simulink model "mapp_4_fir_4_str"  (R2018b)
settings: Solver=ode45  StartTime=0.0  StopTime=200  RelTol=1e-3  EnableMultiTasking=on
undefined symbols (not defined in the file or in its folder): CMD_ci_Re_0, CMD_ci_Re_21, CMD_ci_str_0, CMD_ci_str_1, CMD_ci_str_10, CMD_ci_str_11, CMD_ci_str_12, CMD_ci_str_13, CMD_ci_str_14, CMD_ci_str_15, CMD_ci_str_16, CMD_ci_str_17, CMD_ci_str_18, CMD_ci_str_19, CMD_ci_str_2, CMD_ci_str_20, CMD_ci_str_21, CMD_ci_str_3, CMD_ci_str_4, CMD_ci_str_5, CMD_ci_str_6, CMD_ci_str_7, CMD_ci_str_8, CMD_ci_str_9, CMD_decr_0, CMD_deka_down, CMD_deka_up, CMD_fb, CMD_FB_mult, CMD_Firprg_0, CMD_Firprg_1, CMD_gain, CMD_ind_mult, CMD_ind_mult_1, CMD_ind_mult_2, CMD_ind_mult_3, CMD_ind_mult_4, CMD_ind_stuk, CMD_ind_vol, CMD_ind_vol_1, CMD_ind_vol_2, CMD_ind_vol_3, CMD_ind_vol_4, CMD_init_dac, CMD_init_sw, CMD_molot_string, CMD_nl, CMD_nl_sl, CMD_omega_0, CMD_out_vol, CMD_param_0, CMD_param_5, CMD_pedal, CMD_reset, CMD_rst, CMD_shape_0, CMD_step_down, CMD_step_up, CMD_str_svertk, ind_mult_0 ... (+10)
libraries: xbsIndex_r4 x3300
(part 5 of 16)

== system mapp_4_fir_4_str/MUX0/ci_re_21 ==
  addr : Inport
  m_data : Inport  Port=2
  m_addr : Inport  Port=3
  m_en : Inport  Port=4
  Convert2 : xbsIndex_r4/Convert  gui_display_data_type=Floating-point  arith_type=Floating-point  n_bits=16  bin_pt=14  float_type=Single  exp_bits=8  fraction_bits=24  quantization=Truncate  overflow=Wrap  en=off  latency=6  pipeline=off  dbl_ovrd=off  block_type=convert
  Delay{1..5} (5 alike) : xbsIndex_r4/Delay  rst=off  infoeditControl=Selection of Reset will increase slice count due to use of real FFs and instead of SRLs  en=off  latency=1  reg_retiming=off  dbl_ovrd=off  block_type=delay
  Mux1 : xbsIndex_r4/Mux  inputs=2  en=off  latency=0  precision=Full  arith_type=Unsigned  n_bits=16  bin_pt=14  quantization=Truncate  overflow=Wrap  dbl_ovrd=off  block_type=mux
  Reinterpret9 : xbsIndex_r4/Reinterpret  force_arith_type=on  arith_type=Floating-point  force_bin_pt=on  bin_pt=24  block_type=reinterpret
  Relational14 : xbsIndex_r4/Relational  mode=a=b  op_type=Bool  en=off  latency=0  dbl_ovrd=off  block_type=relational
  Single Port RAM2 : xbsIndex_r4/Single Port RAM  depth=1024  initVector=Res1  distributed_mem=Block RAM  write_mode=Read After Write  rst=off  init_reg=0  en=off  latency=1  optimize=Area  dbl_ovrd=off  block_type=spram
  re_0 : xbsIndex_r4/Constant  const=CMD_ci_Re_21  gui_display_data_type=Fixed-point  arith_type=Unsigned  n_bits=8  bin_pt=0  preci_type=Single  exp_width=8  frac_width=24  explicit_period=on  period=1  equ=P=C  opselect=C  inp2=PCIN>>17  opr=+  inp1=P  carry=CIN  dbl_ovrd=off  block_type=constant
      settings: block_version=VER_STRING_GOES_HERE
  Out : Outport
  wires:
  Delay5/1 -> Single Port RAM2/3, Mux1/1
  Delay1/1 -> Single Port RAM2/2
  Delay4/1 -> Out/1
  Single Port RAM2/1 -> Delay2/1
  Convert2/1 -> Delay4/1
  Delay2/1 -> Reinterpret9/1
  Reinterpret9/1 -> Delay3/1
  Delay3/1 -> Convert2/1
  Mux1/1 -> Single Port RAM2/1
  re_0/1 -> Relational14/2
  Relational14/1 -> Delay5/1
  addr/1 -> Mux1/2
  m_en/1 -> Relational14/1
  m_addr/1 -> Mux1/3
  m_data/1 -> Delay1/1

== system mapp_4_fir_4_str/Mid_Graph2/Exp ==
  note: w5
  Addr_ind_vol : Inport
  Force_vol_sel : Inport  Port=2
  Addr0 : Inport  Port=3
  m_data : Inport  Port=4
  m_addr : Inport  Port=5
  m_en : Inport  Port=6
  Constant3 : xbsIndex_r4/Constant  const=0  gui_display_data_type=Fixed-point  arith_type=Unsigned  n_bits=7  bin_pt=0  preci_type=Single  exp_width=8  frac_width=24  explicit_period=on  period=1  equ=P=C  opselect=C  inp2=PCIN>>17  opr=+  inp1=P  carry=CIN  dbl_ovrd=off  block_type=constant
      settings: block_version=VER_STRING_GOES_HERE
  Convert1 : xbsIndex_r4/Convert  gui_display_data_type=Floating-point  arith_type=Floating-point  n_bits=16  bin_pt=14  float_type=Single  exp_bits=8  fraction_bits=24  quantization=Truncate  overflow=Wrap  en=off  latency=0  pipeline=off  dbl_ovrd=off  block_type=convert
  Convert2 : xbsIndex_r4/Convert  gui_display_data_type=Floating-point  arith_type=Floating-point  n_bits=16  bin_pt=14  float_type=Single  exp_bits=8  fraction_bits=24  quantization=Truncate  overflow=Wrap  en=off  latency=0  pipeline=off  dbl_ovrd=off  block_type=convert
  Convert6 : xbsIndex_r4/Convert  gui_display_data_type=Floating-point  arith_type=Floating-point  n_bits=16  bin_pt=14  float_type=Single  exp_bits=8  fraction_bits=24  quantization=Truncate  overflow=Wrap  en=off  latency=0  pipeline=off  dbl_ovrd=off  block_type=convert
  Convert9 : xbsIndex_r4/Convert  gui_display_data_type=Fixed-point  arith_type=Unsigned  n_bits=24  bin_pt=0  float_type=Single  exp_bits=8  fraction_bits=24  quantization=Truncate  overflow=Wrap  en=off  latency=0  pipeline=off  dbl_ovrd=off  block_type=convert
  Mult : xbsIndex_r4/Mult  precision=Full  arith_type="Signed  (2's comp)"  n_bits=16  bin_pt=14  quantization=Truncate  overflow=Wrap  en=off  latency=6  use_behavioral_HDL=off  opt=Speed  use_embedded=on  optimum_pipeline=off  pipeline=on  dbl_ovrd=off  use_rpm=on  placement_style=Triangular  block_type=mult
  Mult1 : xbsIndex_r4/Mult  precision=Full  arith_type="Signed  (2's comp)"  n_bits=16  bin_pt=14  quantization=Truncate  overflow=Wrap  en=off  latency=6  use_behavioral_HDL=off  opt=Speed  use_embedded=on  optimum_pipeline=off  pipeline=on  dbl_ovrd=off  use_rpm=on  placement_style=Triangular  block_type=mult
  Relational16 : xbsIndex_r4/Relational  mode=a=b  op_type=Bool  en=off  latency=0  dbl_ovrd=off  block_type=relational
  Scope2 : Scope  NumInputPorts=9
  Scope3 : Scope  NumInputPorts=9
  const : xbsIndex_r4/Constant  const=0  gui_display_data_type=Fixed-point  arith_type=Unsigned  n_bits=7  bin_pt=0  preci_type=Single  exp_width=8  frac_width=24  explicit_period=on  period=1  equ=P=C  opselect=C  inp2=PCIN>>17  opr=+  inp1=P  carry=CIN  dbl_ovrd=off  block_type=constant
      settings: block_version=VER_STRING_GOES_HERE
  exp-mashinka : Subsystem
  ind_tails : Subsystem
  ind_vol : Subsystem
  z1 : xbsIndex_r4/Delay  rst=off  infoeditControl=Selection of Reset will increase slice count due to use of real FFs and instead of SRLs  en=off  latency=66  reg_retiming=on  dbl_ovrd=off  block_type=delay
      settings: block_version=8.2-EVAL
  z{2..3,5..7} (5 alike) : xbsIndex_r4/Delay  rst=off  infoeditControl=Selection of Reset will increase slice count due to use of real FFs and instead of SRLs  en=off  latency=1  reg_retiming=on  dbl_ovrd=off  block_type=delay
      settings: block_version=8.2-EVAL
  z4 : xbsIndex_r4/Delay  rst=off  infoeditControl=Selection of Reset will increase slice count due to use of real FFs and instead of SRLs  en=off  latency=66 + 7  reg_retiming=on  dbl_ovrd=off  block_type=delay
      settings: block_version=8.2-EVAL
  z53 : xbsIndex_r4/Delay  rst=off  infoeditControl=Selection of Reset will increase slice count due to use of real FFs and instead of SRLs  en=off  latency=9  reg_retiming=on  dbl_ovrd=off  block_type=delay
      settings: block_version=8.2-EVAL
  z8 : xbsIndex_r4/Delay  rst=off  infoeditControl=Selection of Reset will increase slice count due to use of real FFs and instead of SRLs  en=off  latency=2  reg_retiming=on  dbl_ovrd=off  block_type=delay
      settings: block_version=8.2-EVAL
  FF : Outport
  Stuk : Outport  Port=2
  wires:
  z7/1 -> Mult1/1
  z6/1 -> Stuk/1
  Mult1/1 -> z6/1
  z5/1 -> Mult1/2
  ind_tails/1(Out1) -> z4/1
  z4/1 -> z5/1
  z3/1 -> FF/1
  Mult/1 -> z7/1, Convert2/1, z3/1
  Convert2/1 -> Scope3/3
  Convert1/1 -> Scope3/2
  exp-mashinka/1(Out) -> Convert6/1, Mult/1
  z2/1 -> Mult/2, Convert1/1
  z1/1 -> z2/1
  Convert6/1 -> Scope3/1
  ind_vol/1(Out1) -> z1/1
  Relational16/1 -> z53/1
  const/1 -> Relational16/2
  m_addr/1 -> exp-mashinka/3(m_addr), ind_vol/3(m_addr), ind_tails/3(m_addr)
  m_data/1 -> Convert9/1, exp-mashinka/2(m_data), ind_vol/2(dat_in), ind_tails/2(dat_in)
  m_en/1 -> exp-mashinka/4(m_en), ind_vol/4(m_en), ind_tails/4(m_en)
  z8/1 -> exp-mashinka/1(Force_vol), ind_vol/5(force_vol), ind_tails/5(force_vol)
  Addr_ind_vol/1 -> exp-mashinka/5(Addr_ind_vol), ind_vol/1(addr_ind_vol), ind_tails/1(addr_ind_vol), Scope2/1
  Addr0/1 -> exp-mashinka/6(Addr_sync), Scope2/3
  Force_vol_sel/1 -> Relational16/1, Scope2/2, z8/1

== system mapp_4_fir_4_str/Mid_Graph2/ind_mult ==
  addr : Inport
  dat_in : Inport  Port=2
  addr_prg : Inport  Port=3
  prg_en : Inport  Port=4
  force_vol : Inport  Port=5
  AddSub5 : xbsIndex_r4/AddSub  mode=Subtraction  use_carryin=off  use_carryout=off  en=off  latency=2  precision=Full  arith_type="Signed  (2's comp)"  n_bits=24  bin_pt=0  quantization=Truncate  overflow=Wrap  use_behavioral_HDL=off  hw_selection=Fabric  pipelined=off  dbl_ovrd=off  block_type=addsub
  AddSub6 : xbsIndex_r4/AddSub  mode=Addition  use_carryin=off  use_carryout=off  en=off  latency=2  precision=Full  arith_type=Unsigned  n_bits=24  bin_pt=0  quantization=Truncate  overflow=Wrap  use_behavioral_HDL=off  hw_selection=Fabric  pipelined=off  dbl_ovrd=off  block_type=addsub
  Constant : xbsIndex_r4/Constant  const=4  gui_display_data_type=Fixed-point  arith_type=Unsigned  n_bits=3  bin_pt=0  preci_type=Single  exp_width=8  frac_width=24  explicit_period=off  period=1  equ=P=C  opselect=C  inp2=PCIN>>17  opr=+  inp1=P  carry=CIN  dbl_ovrd=off  block_type=constant
  Constant1 : xbsIndex_r4/Constant  const=0  gui_display_data_type=Fixed-point  arith_type=Unsigned  n_bits=24  bin_pt=0  preci_type=Single  exp_width=8  frac_width=24  explicit_period=on  period=1  equ=P=C  opselect=C  inp2=PCIN>>17  opr=+  inp1=P  carry=CIN  dbl_ovrd=off  block_type=constant
      settings: block_version=VER_STRING_GOES_HERE
  Constant10 : xbsIndex_r4/Constant  const=0  gui_display_data_type=Fixed-point  arith_type=Unsigned  n_bits=24  bin_pt=0  preci_type=Single  exp_width=8  frac_width=24  explicit_period=on  period=1  equ=P=C  opselect=C  inp2=PCIN>>17  opr=+  inp1=P  carry=CIN  dbl_ovrd=off  block_type=constant
      settings: block_version=VER_STRING_GOES_HERE
  Constant2 : xbsIndex_r4/Constant  const=4  gui_display_data_type=Fixed-point  arith_type=Unsigned  n_bits=3  bin_pt=0  preci_type=Single  exp_width=8  frac_width=24  explicit_period=on  period=1  equ=P=C  opselect=C  inp2=PCIN>>17  opr=+  inp1=P  carry=CIN  dbl_ovrd=off  block_type=constant
      settings: block_version=VER_STRING_GOES_HERE
  Constant3 : xbsIndex_r4/Constant  const=3  gui_display_data_type=Fixed-point  arith_type=Unsigned  n_bits=3  bin_pt=0  preci_type=Single  exp_width=8  frac_width=24  explicit_period=off  period=1  equ=P=C  opselect=C  inp2=PCIN>>17  opr=+  inp1=P  carry=CIN  dbl_ovrd=off  block_type=constant
  Constant4 : xbsIndex_r4/Constant  const=2  gui_display_data_type=Fixed-point  arith_type=Unsigned  n_bits=3  bin_pt=0  preci_type=Single  exp_width=8  frac_width=24  explicit_period=off  period=1  equ=P=C  opselect=C  inp2=PCIN>>17  opr=+  inp1=P  carry=CIN  dbl_ovrd=off  block_type=constant
  Constant5 : xbsIndex_r4/Constant  const=1  gui_display_data_type=Fixed-point  arith_type=Unsigned  n_bits=3  bin_pt=0  preci_type=Single  exp_width=8  frac_width=24  explicit_period=off  period=1  equ=P=C  opselect=C  inp2=PCIN>>17  opr=+  inp1=P  carry=CIN  dbl_ovrd=off  block_type=constant
  Constant6 : xbsIndex_r4/Constant  const=0  gui_display_data_type=Fixed-point  arith_type=Unsigned  n_bits=3  bin_pt=0  preci_type=Single  exp_width=8  frac_width=24  explicit_period=off  period=1  equ=P=C  opselect=C  inp2=PCIN>>17  opr=+  inp1=P  carry=CIN  dbl_ovrd=off  block_type=constant
  Convert5 : xbsIndex_r4/Convert  gui_display_data_type=Fixed-point  arith_type=Unsigned  n_bits=3  bin_pt=0  float_type=Single  exp_bits=8  fraction_bits=24  quantization=Truncate  overflow=Wrap  en=off  latency=0  pipeline=off  dbl_ovrd=off  block_type=convert
  Logical{,1..4} (5 alike) : xbsIndex_r4/Logical  logical_function=AND  inputs=2  en=off  latency=1  precision=Full  arith_type=Unsigned  n_bits=16  bin_pt=0  align_bp=on  dbl_ovrd=off  block_type=logical
  Mult3 : xbsIndex_r4/Mult  precision=Full  arith_type="Signed  (2's comp)"  n_bits=16  bin_pt=14  quantization=Truncate  overflow=Wrap  en=off  latency=3  use_behavioral_HDL=off  opt=Speed  use_embedded=on  optimum_pipeline=off  pipeline=on  dbl_ovrd=off  use_rpm=on  placement_style=Triangular  block_type=mult
  Mux{1,10..14} (6 alike) : xbsIndex_r4/Mux  inputs=2  en=off  latency=0  precision=Full  arith_type=Unsigned  n_bits=16  bin_pt=14  quantization=Truncate  overflow=Wrap  dbl_ovrd=off  block_type=mux
  Mux2 : xbsIndex_r4/Mux  inputs=5  en=off  latency=1  precision=Full  arith_type=Unsigned  n_bits=16  bin_pt=14  quantization=Truncate  overflow=Wrap  dbl_ovrd=off  block_type=mux
  Mux3 : xbsIndex_r4/Mux  inputs=5  en=off  latency=1  precision=Full  arith_type=Unsigned  n_bits=16  bin_pt=14  quantization=Truncate  overflow=Wrap  dbl_ovrd=off  block_type=mux
  RSlice1 : xbsIndex_r4/Slice  nbits=3  boolean_output=off  mode=Upper Bit Location + Width  bit1=0  base1=MSB of Input  bit0=0  base0=LSB of Input  dbl_ovrd=off  block_type=slice
      settings: block_version=VER_STRING_GOES_HERE
  RSlice7 : xbsIndex_r4/Slice  nbits=7  boolean_output=off  mode=Lower Bit Location + Width  bit1=0  base1=MSB of Input  bit0=0  base0=LSB of Input  dbl_ovrd=off  block_type=slice
      settings: block_version=VER_STRING_GOES_HERE
  Relational{1..5,16..17} (7 alike) : xbsIndex_r4/Relational  mode=a=b  op_type=Bool  en=off  latency=0  dbl_ovrd=off  block_type=relational
  Scope1 : Scope  NumInputPorts=8
  Scope2 : Scope  NumInputPorts=10
  Scope3 : Scope  NumInputPorts=10
  Scope4 : Scope  NumInputPorts=10
  Shift2 : xbsIndex_r4/Shift  shift_dir=Right  shift_bits=5  en=off  latency=0  precision=Full  arith_type="Signed  (2's comp)"  n_bits=16  bin_pt=14  quantization=Truncate  overflow=Wrap  dbl_ovrd=off  block_type=shift
  Single Port RAM5 : xbsIndex_r4/Single Port RAM  depth=96  initVector=ind_mult_4*ind_mult_multiplier  distributed_mem=Block RAM  write_mode=Read After Write  rst=off  init_reg=0  en=off  latency=1  optimize=Area  dbl_ovrd=off  block_type=spram
  Single Port RAM6 : xbsIndex_r4/Single Port RAM  depth=96  initVector=ind_mult_3*ind_mult_multiplier  distributed_mem=Block RAM  write_mode=Read After Write  rst=off  init_reg=0  en=off  latency=1  optimize=Area  dbl_ovrd=off  block_type=spram
  Single Port RAM7 : xbsIndex_r4/Single Port RAM  depth=96  initVector=ind_mult_2*ind_mult_multiplier  distributed_mem=Block RAM  write_mode=Read After Write  rst=off  init_reg=0  en=off  latency=1  optimize=Area  dbl_ovrd=off  block_type=spram
  Single Port RAM8 : xbsIndex_r4/Single Port RAM  depth=96  initVector=ind_mult_1*ind_mult_multiplier  distributed_mem=Block RAM  write_mode=Read After Write  rst=off  init_reg=0  en=off  latency=1  optimize=Area  dbl_ovrd=off  block_type=spram
  Single Port RAM9 : xbsIndex_r4/Single Port RAM  depth=96  initVector=ind_mult_0*ind_mult_multiplier  distributed_mem=Block RAM  write_mode=Read After Write  rst=off  init_reg=0  en=off  latency=1  optimize=Area  dbl_ovrd=off  block_type=spram
  Slice1 : xbsIndex_r4/Slice  nbits=5  boolean_output=off  mode=Lower Bit Location + Width  bit1=0  base1=LSB of Input  bit0=0  base0=LSB of Input  dbl_ovrd=off  block_type=slice
  Slice3 : xbsIndex_r4/Slice  nbits=2  boolean_output=off  mode=Upper Bit Location + Width  bit1=0  base1=MSB of Input  bit0=0  base0=LSB of Input  dbl_ovrd=off  block_type=slice
  const : xbsIndex_r4/Constant  const=0  gui_display_data_type=Fixed-point  arith_type=Unsigned  n_bits=7  bin_pt=0  preci_type=Single  exp_width=8  frac_width=24  explicit_period=on  period=1  equ=P=C  opselect=C  inp2=PCIN>>17  opr=+  inp1=P  carry=CIN  dbl_ovrd=off  block_type=constant
      settings: block_version=VER_STRING_GOES_HERE
  ind_mult : xbsIndex_r4/Constant  const=CMD_ind_mult  gui_display_data_type=Fixed-point  arith_type=Unsigned  n_bits=8  bin_pt=0  preci_type=Single  exp_width=8  frac_width=24  explicit_period=on  period=1  equ=P=C  opselect=C  inp2=PCIN>>17  opr=+  inp1=P  carry=CIN  dbl_ovrd=off  block_type=constant
      settings: block_version=VER_STRING_GOES_HERE
  x : xbsIndex_r4/Constant  const=8000000  gui_display_data_type=Fixed-point  arith_type=Unsigned  n_bits=24  bin_pt=0  preci_type=Single  exp_width=8  frac_width=24  explicit_period=on  period=1  equ=P=C  opselect=C  inp2=PCIN>>17  opr=+  inp1=P  carry=CIN  dbl_ovrd=off  block_type=constant
      settings: block_version=VER_STRING_GOES_HERE
  z1 : xbsIndex_r4/Delay  rst=off  infoeditControl=Selection of Reset will increase slice count due to use of real FFs and instead of SRLs  en=off  latency=3  reg_retiming=on  dbl_ovrd=off  block_type=delay
      settings: block_version=8.2-EVAL
  z{2,5..13,15} (11 alike) : xbsIndex_r4/Delay  rst=off  infoeditControl=Selection of Reset will increase slice count due to use of real FFs and instead of SRLs  en=off  latency=1  reg_retiming=on  dbl_ovrd=off  block_type=delay
      settings: block_version=8.2-EVAL
  z14 : xbsIndex_r4/Delay  rst=off  infoeditControl=Selection of Reset will increase slice count due to use of real FFs and instead of SRLs  en=off  latency=2  reg_retiming=on  dbl_ovrd=off  block_type=delay
      settings: block_version=8.2-EVAL
  z3 : xbsIndex_r4/Delay  rst=off  infoeditControl=Selection of Reset will increase slice count due to use of real FFs and instead of SRLs  en=off  latency=4  reg_retiming=on  dbl_ovrd=off  block_type=delay
      settings: block_version=8.2-EVAL
  z4 : xbsIndex_r4/Delay  rst=off  infoeditControl=Selection of Reset will increase slice count due to use of real FFs and instead of SRLs  en=off  latency=2  reg_retiming=on  dbl_ovrd=off  block_type=delay
      settings: block_version=8.2-EVAL
  Out1 : Outport
  wires:
  z1/1 -> Mult3/2, Scope1/5
  Mux1/1 -> Scope3/1, Mux2/1, Mux3/1
  z15/1 -> Mux3/2
  z13/1 -> Scope3/2, Mux2/2, Mux3/3
  z12/1 -> Mux3/4, Scope3/3, Mux2/3
  z11/1 -> Scope3/4, Mux2/4, Mux3/5
  z10/1 -> Scope3/5, Mux2/5
  AddSub6/1 -> Out1/1, Scope1/8
  z3/1 -> AddSub6/2, Scope1/7
  z14/1 -> z3/1
  z2/1 -> AddSub6/1, Scope1/6
  Mult3/1 -> z2/1
  Slice1/1 -> z1/1
  Shift2/1 -> Mult3/1, Scope1/4
  AddSub5/1 -> Shift2/1, Scope1/3
  Mux3/1 -> AddSub5/2, Scope1/2, Scope3/7, z14/1
  Mux2/1 -> AddSub5/1, Scope1/1, Scope3/6
  Constant1/1 -> Mux3/6
  Constant10/1 -> Mux2/6
  Slice3/1 -> Convert5/1
  Convert5/1 -> Mux1/2
  Relational16/1 -> Mux1/1
  Constant2/1 -> Mux1/3
  const/1 -> Relational16/2
  Single Port RAM5/1 -> z10/1, Scope2/2
  Single Port RAM6/1 -> z11/1, Scope2/4
  Single Port RAM7/1 -> z12/1
  Single Port RAM9/1 -> z15/1
  Single Port RAM8/1 -> z13/1
  force_vol/1 -> Slice3/1, Slice1/1, Relational16/1
  prg_en/1 -> Relational17/1
  addr_prg/1 -> RSlice7/1, RSlice1/1
  Mux14/1 -> Single Port RAM9/1
  Logical4/1 -> Mux14/1, Single Port RAM9/3
  addr/1 -> z4/1
  Mux12/1 -> Single Port RAM7/1
  Mux13/1 -> Single Port RAM8/1
  Mux11/1 -> Single Port RAM6/1, Scope2/3
  Logical2/1 -> Mux12/1, Single Port RAM7/3
  ind_mult/1 -> Relational17/2
  Logical1/1 -> Mux11/1, Single Port RAM6/3
  Logical/1 -> Single Port RAM5/3, Mux10/1
  Logical3/1 -> Single Port RAM8/3, Mux13/1
  Mux10/1 -> Single Port RAM5/1, Scope2/1
  dat_in/1 -> Single Port RAM5/2, Single Port RAM8/2, Single Port RAM9/2, Single Port RAM7/2, Single Port RAM6/2
  z4/1 -> z5/1, z6/1, z8/1, z9/1, z7/1
  z5/1 -> Mux10/2
  z6/1 -> Mux11/2
  z7/1 -> Mux12/2
  z8/1 -> Mux13/2
  z9/1 -> Mux14/2
  RSlice7/1 -> Mux10/3, Mux13/3, Mux14/3, Mux12/3, Mux11/3
  RSlice1/1 -> Relational2/1, Relational3/1, Relational4/1, Relational5/1, Relational1/1
  Constant/1 -> Relational1/2
  Constant3/1 -> Relational2/2
  Constant4/1 -> Relational3/2
  Constant5/1 -> Relational4/2
  Constant6/1 -> Relational5/2
  Relational17/1 -> Logical1/1, Logical2/1, Logical3/1, Logical4/1, Logical/1
  Relational1/1 -> Logical/2
  Relational2/1 -> Logical1/2
  Relational3/1 -> Logical2/2
  Relational4/1 -> Logical3/2
  Relational5/1 -> Logical4/2

== system mapp_4_fir_4_str/Mid_Graph2/noise_gen ==
  AddSub : xbsIndex_r4/AddSub  mode=Addition  use_carryin=off  use_carryout=off  en=off  latency=1  precision=Full  arith_type=Unsigned  n_bits=16  bin_pt=14  quantization=Truncate  overflow=Wrap  use_behavioral_HDL=off  hw_selection=Fabric  pipelined=off  dbl_ovrd=off  block_type=addsub
  Counter : xbsIndex_r4/Counter  cnt_type=Free Running  cnt_to=Inf  operation=Up  start_count=0  cnt_by_val=1  arith_type=Unsigned  n_bits=16  bin_pt=0  load_pin=off  rst=off  en=on  explicit_period=on  period=1  use_behavioral_HDL=off  implementation=Fabric  dbl_ovrd=off  block_type=counter
  Counter2 : xbsIndex_r4/Counter  cnt_type=Count Limited  cnt_to=rom_length*8 - 1  operation=Up  start_count=0  cnt_by_val=1  arith_type=Unsigned  n_bits=16  bin_pt=0  load_pin=off  rst=off  en=off  explicit_period=on  period=1  use_behavioral_HDL=off  implementation=Fabric  dbl_ovrd=off  block_type=counter
  Counter4 : xbsIndex_r4/Counter  cnt_type=Count Limited  cnt_to=rom_length-1  operation=Up  start_count=0  cnt_by_val=1  arith_type=Unsigned  n_bits=13  bin_pt=0  load_pin=off  rst=off  en=on  explicit_period=on  period=1  use_behavioral_HDL=off  implementation=Fabric  dbl_ovrd=off  block_type=counter
  Counter5 : xbsIndex_r4/Counter  cnt_type=Count Limited  cnt_to=rom_length - 2  operation=Up  start_count=0  cnt_by_val=1  arith_type=Unsigned  n_bits=13  bin_pt=0  load_pin=off  rst=off  en=on  explicit_period=on  period=1  use_behavioral_HDL=off  implementation=Fabric  dbl_ovrd=off  block_type=counter
  Dual Port RAM : xbsIndex_r4/Dual Port RAM  depth=rom_length  initVector=noise_0  distributed_mem=Block RAM  init_a=0  init_b=0  rst_a=off  rst_b=off  en_a=off  en_b=off  latency=1  write_mode_A=Read After Write  write_mode_B=Read After Write  optimize=Speed  dbl_ovrd=off  block_type=dpram
  Dual Port RAM1 : xbsIndex_r4/Dual Port RAM  depth=rom_length  initVector=noise_1  distributed_mem=Block RAM  init_a=0  init_b=0  rst_a=off  rst_b=off  en_a=off  en_b=off  latency=2  write_mode_A=Read After Write  write_mode_B=Read After Write  optimize=Speed  dbl_ovrd=off  block_type=dpram
  Dual Port RAM3 : xbsIndex_r4/Dual Port RAM  depth=rom_length  initVector=noise_2  distributed_mem=Block RAM  init_a=0  init_b=0  rst_a=off  rst_b=off  en_a=off  en_b=off  latency=2  write_mode_A=Read After Write  write_mode_B=Read After Write  optimize=Speed  dbl_ovrd=off  block_type=dpram
  Dual Port RAM4 : xbsIndex_r4/Dual Port RAM  depth=rom_length  initVector=noise_3  distributed_mem=Block RAM  init_a=0  init_b=0  rst_a=off  rst_b=off  en_a=off  en_b=off  latency=2  write_mode_A=Read After Write  write_mode_B=Read After Write  optimize=Speed  dbl_ovrd=off  block_type=dpram
  Dual Port RAM5 : xbsIndex_r4/Dual Port RAM  depth=rom_length  initVector=noise_4  distributed_mem=Block RAM  init_a=0  init_b=0  rst_a=off  rst_b=off  en_a=off  en_b=off  latency=2  write_mode_A=Read After Write  write_mode_B=Read After Write  optimize=Speed  dbl_ovrd=off  block_type=dpram
  Dual Port RAM6 : xbsIndex_r4/Dual Port RAM  depth=rom_length  initVector=noise_5  distributed_mem=Block RAM  init_a=0  init_b=0  rst_a=off  rst_b=off  en_a=off  en_b=off  latency=2  write_mode_A=Read After Write  write_mode_B=Read After Write  optimize=Speed  dbl_ovrd=off  block_type=dpram
  Dual Port RAM7 : xbsIndex_r4/Dual Port RAM  depth=rom_length  initVector=noise_6  distributed_mem=Block RAM  init_a=0  init_b=0  rst_a=off  rst_b=off  en_a=off  en_b=off  latency=2  write_mode_A=Read After Write  write_mode_B=Read After Write  optimize=Speed  dbl_ovrd=off  block_type=dpram
  Dual Port RAM8 : xbsIndex_r4/Dual Port RAM  depth=rom_length  initVector=noise_7  distributed_mem=Block RAM  init_a=0  init_b=0  rst_a=off  rst_b=off  en_a=off  en_b=off  latency=2  write_mode_A=Read After Write  write_mode_B=Read After Write  optimize=Speed  dbl_ovrd=off  block_type=dpram
  Mux : xbsIndex_r4/Mux  inputs=8  en=off  latency=1  precision=Full  arith_type=Unsigned  n_bits=16  bin_pt=14  quantization=Truncate  overflow=Wrap  dbl_ovrd=off  block_type=mux
  Mux1 : xbsIndex_r4/Mux  inputs=8  en=off  latency=1  precision=Full  arith_type=Unsigned  n_bits=16  bin_pt=14  quantization=Truncate  overflow=Wrap  dbl_ovrd=off  block_type=mux
  Relational3 : xbsIndex_r4/Relational  mode=a=b  op_type=Bool  en=off  latency=1  dbl_ovrd=off  block_type=relational
  Slice : xbsIndex_r4/Slice  nbits=3  boolean_output=off  mode=Upper Bit Location + Width  bit1=0  base1=MSB of Input  bit0=0  base0=LSB of Input  dbl_ovrd=off  block_type=slice
  q1 : xbsIndex_r4/Constant  const=0  gui_display_data_type=Fixed-point  arith_type=Unsigned  n_bits=10  bin_pt=0  preci_type=Single  exp_width=8  frac_width=24  explicit_period=on  period=1  equ=P=C  opselect=C  inp2=PCIN>>17  opr=+  inp1=P  carry=CIN  dbl_ovrd=off  block_type=constant
      settings: block_version=VER_STRING_GOES_HERE
  q{4,6,10..11,13,15,17,19} (8 alike) : xbsIndex_r4/Constant  const=0  gui_display_data_type=Boolean  arith_type=Boolean  n_bits=24  bin_pt=23  preci_type=Single  exp_width=8  frac_width=24  explicit_period=on  period=1  equ=P=C  opselect=C  inp2=PCIN>>17  opr=+  inp1=P  carry=CIN  dbl_ovrd=off  block_type=constant
      settings: block_version=VER_STRING_GOES_HERE
  q{3,5,9,12,14,16,18,20} (8 alike) : xbsIndex_r4/Constant  const=0  gui_display_data_type=Fixed-point  arith_type=Signed (2's comp)  n_bits=24  bin_pt=23  preci_type=Single  exp_width=8  frac_width=24  explicit_period=on  period=1  equ=P=C  opselect=C  inp2=PCIN>>17  opr=+  inp1=P  carry=CIN  dbl_ovrd=off  block_type=constant
      settings: block_version=VER_STRING_GOES_HERE
  q2 : xbsIndex_r4/Constant  const=1  gui_display_data_type=Boolean  arith_type=Boolean  n_bits=10  bin_pt=0  preci_type=Single  exp_width=8  frac_width=24  explicit_period=on  period=1  equ=P=C  opselect=C  inp2=PCIN>>17  opr=+  inp1=P  carry=CIN  dbl_ovrd=off  block_type=constant
      settings: block_version=VER_STRING_GOES_HERE
  z{1..18,26..28} (21 alike) : xbsIndex_r4/Delay  rst=off  infoeditControl=Selection of Reset will increase slice count due to use of real FFs and instead of SRLs  en=off  latency=1  reg_retiming=on  dbl_ovrd=off  block_type=delay
      settings: block_version=8.2-EVAL
  Out2 : Outport
  wires:
  z5/1 -> Mux/5
  z17/1 -> Mux1/2
  Slice/1 -> Mux/1, Mux1/1
  z1/1 -> Mux/3
  q11/1 -> Dual Port RAM4/6, Dual Port RAM4/3
  Dual Port RAM1/2 -> z2/1
  Dual Port RAM1/1 -> z1/1
  Dual Port RAM4/2 -> z6/1
  Dual Port RAM5/1 -> z7/1
  Dual Port RAM8/1 -> z18/1
  Dual Port RAM4/1 -> z5/1
  Dual Port RAM6/2 -> z10/1
  q4/1 -> Dual Port RAM/6, Dual Port RAM/3
  Dual Port RAM/2 -> z17/1
  z16/1 -> Mux/2
  Mux1/1 -> z15/1
  z14/1 -> AddSub/1
  z11/1 -> Mux1/8
  z3/1 -> Mux/4
  z15/1 -> AddSub/2
  Dual Port RAM7/1 -> z12/1
  Dual Port RAM3/2 -> z4/1
  q15/1 -> Dual Port RAM6/6, Dual Port RAM6/3
  z8/1 -> Mux1/6
  q13/1 -> Dual Port RAM5/3, Dual Port RAM5/6
  Dual Port RAM7/2 -> z11/1
  z9/1 -> Mux/7
  z12/1 -> Mux/8
  z4/1 -> Mux1/4
  q10/1 -> Dual Port RAM3/3, Dual Port RAM3/6
  Dual Port RAM5/2 -> z8/1
  z10/1 -> Mux1/7
  z18/1 -> Mux/9
  q14/1 -> Dual Port RAM5/5, Dual Port RAM5/2
  q1/1 -> Relational3/2
  z28/1 -> Relational3/1
  q19/1 -> Dual Port RAM8/6, Dual Port RAM8/3
  Counter/1 -> Slice/1
  z13/1 -> Mux1/9
  q5/1 -> Dual Port RAM1/5, Dual Port RAM1/2
  Dual Port RAM8/2 -> z13/1
  AddSub/1 -> Out2/1
  Relational3/1 -> Counter4/1, Counter/1, Counter5/1
  q9/1 -> Dual Port RAM3/5, Dual Port RAM3/2
  Counter4/1 -> z26/1
  q3/1 -> Dual Port RAM/2, Dual Port RAM/5
  z26/1 -> Dual Port RAM/1, Dual Port RAM8/1, Dual Port RAM7/1, Dual Port RAM6/1, Dual Port RAM5/1, Dual Port RAM4/1, Dual Port RAM3/1, Dual Port RAM1/1
  Dual Port RAM/1 -> z16/1
  q6/1 -> Dual Port RAM1/3, Dual Port RAM1/6
  q20/1 -> Dual Port RAM8/2, Dual Port RAM8/5
  Mux/1 -> z14/1
  q16/1 -> Dual Port RAM6/2, Dual Port RAM6/5
  q18/1 -> Dual Port RAM7/5, Dual Port RAM7/2
  Dual Port RAM6/1 -> z9/1
  Counter5/1 -> z27/1
  z2/1 -> Mux1/3
  q17/1 -> Dual Port RAM7/3, Dual Port RAM7/6
  Dual Port RAM3/1 -> z3/1
  Counter2/1 -> z28/1
  z6/1 -> Mux1/5
  q12/1 -> Dual Port RAM4/2, Dual Port RAM4/5
  z7/1 -> Mux/6
  z27/1 -> Dual Port RAM/4, Dual Port RAM8/4, Dual Port RAM7/4, Dual Port RAM6/4, Dual Port RAM5/4, Dual Port RAM4/4, Dual Port RAM3/4, Dual Port RAM1/4

== system mapp_4_fir_4_str/Mid_Graph2/start_delay ==
  Constant4 : xbsIndex_r4/Constant  const=100  gui_display_data_type=Fixed-point  arith_type=Unsigned  n_bits=7  bin_pt=0  preci_type=Single  exp_width=8  frac_width=24  explicit_period=on  period=1  equ=P=C  opselect=C  inp2=PCIN>>17  opr=+  inp1=P  carry=CIN  dbl_ovrd=off  block_type=constant
      settings: block_version=VER_STRING_GOES_HERE
  Constant6 : xbsIndex_r4/Constant  const=0  gui_display_data_type=Boolean  arith_type=Boolean  n_bits=7  bin_pt=0  preci_type=Single  exp_width=8  frac_width=24  explicit_period=on  period=1  equ=P=C  opselect=C  inp2=PCIN>>17  opr=+  inp1=P  carry=CIN  dbl_ovrd=off  block_type=constant
      settings: block_version=VER_STRING_GOES_HERE
  Counter1 : xbsIndex_r4/Counter  cnt_type=Free Running  cnt_to=95  operation=Up  start_count=0  cnt_by_val=1  arith_type=Unsigned  n_bits=7  bin_pt=0  load_pin=off  rst=off  en=on  explicit_period=on  period=1  use_behavioral_HDL=off  implementation=Fabric  use_rpm=off  dbl_ovrd=off  block_type=counter
      settings: block_version=8.2.02
  Register3 : xbsIndex_r4/Register  init=1  rst=off  en=on  dbl_ovrd=off  block_type=register
  Relational3 : xbsIndex_r4/Relational  mode=a>b  op_type=Bool  en=off  latency=0  dbl_ovrd=off  block_type=relational
  Out1 : Outport
  wires:
  Constant4/1 -> Relational3/2
  Counter1/1 -> Relational3/1
  Relational3/1 -> Out1/1, Register3/2
  Constant6/1 -> Register3/1
  Register3/1 -> Counter1/1

== system mapp_4_fir_4_str/Reciever16/Subsystem1 ==
  data : Inport
  en : Inport  Port=2
  clock : Inport  Port=3
  reset : Inport  Port=4
  Concat : xbsIndex_r4/Concat  num_inputs=16  dbl_ovrd=off  block_type=concat
      settings: block_version=8.2-EVAL
  Register{1..15,32} (16 alike) : xbsIndex_r4/Register  init=0  rst=on  en=on  dbl_ovrd=off  block_type=register
      settings: xl_area=[1 1 0 0 0 0 0]  block_version=8.2-EVAL
  Register{64..79} (16 alike) : xbsIndex_r4/Register  init=0  rst=off  en=on  dbl_ovrd=off  block_type=register
      settings: xl_area=[1 1 0 0 0 0 0]  block_version=8.2-EVAL
  Out1 : Outport
  wires:
  Register32/1 -> Concat/16
  Register1/1 -> Concat/15
  Register2/1 -> Concat/14
  Register3/1 -> Concat/13
  Register4/1 -> Concat/12
  Register5/1 -> Concat/11
  Register6/1 -> Concat/10
  Register7/1 -> Concat/9
  Register8/1 -> Concat/8
  Register9/1 -> Concat/7
  Register10/1 -> Concat/6
  Register11/1 -> Concat/5
  Register12/1 -> Concat/4
  Register13/1 -> Concat/3
  Register14/1 -> Concat/2
  Register15/1 -> Concat/1
  reset/1 -> Register15/2, Register14/2, Register13/2, Register12/2, Register11/2, Register10/2, Register9/2, Register8/2, Register7/2, Register6/2, Register5/2, Register4/2, Register3/2, Register2/2, Register1/2, Register32/2
  en/1 -> Register15/3, Register14/3, Register13/3, Register12/3, Register11/3, Register10/3, Register9/3, Register8/3, Register7/3, Register6/3, Register5/3, Register4/3, Register1/3, Register32/3, Register2/3, Register3/3
  Register64/1 -> Register65/1, Register32/1
  data/1 -> Register64/1
  Register65/1 -> Register66/1, Register1/1
  Register66/1 -> Register67/1, Register2/1
  Register67/1 -> Register68/1, Register3/1
  Register68/1 -> Register69/1, Register4/1
  Register69/1 -> Register70/1, Register5/1
  Register70/1 -> Register71/1, Register6/1
  Register71/1 -> Register72/1, Register7/1
  Register72/1 -> Register73/1, Register8/1
  Register73/1 -> Register74/1, Register9/1
  Register74/1 -> Register75/1, Register10/1
  Register75/1 -> Register76/1, Register11/1
  Register76/1 -> Register77/1, Register12/1
  Register77/1 -> Register78/1, Register13/1
  Register78/1 -> Register79/1, Register14/1
  Register79/1 -> Register15/1
  clock/1 -> Register79/2, Register78/2, Register77/2, Register76/2, Register75/2, Register74/2, Register73/2, Register71/2, Register70/2, Register69/2, Register68/2, Register67/2, Register64/2, Register65/2, Register66/2, Register72/2
  Concat/1 -> Out1/1

== system mapp_4_fir_4_str/Reciever16/Z1 ==
  In1 : Inport
  Delay3 : xbsIndex_r4/Delay  rst=off  infoeditControl=Selection of Reset will increase slice count due to use of real FFs and instead of SRLs  en=off  latency=1  reg_retiming=on  dbl_ovrd=off  block_type=delay
      settings: infoedit=Hardware notes: A delay line is a chain, each link of which is an SRL16 followed by a flip-flop. If register retiming is enabled, the delay line is a chain of flip-flops.  xl_area=[1 1 0 0 0 0 0]  block_version=8.2-EVAL
  Inverter : xbsIndex_r4/Inverter  en=off  latency=1  dbl_ovrd=off  block_type=inv
      settings: xl_area=[1 1 0 0 0 0 0]  block_version=8.2-EVAL
  Logical : xbsIndex_r4/Logical  logical_function=XOR  inputs=2  en=off  latency=1  precision=Full  arith_type=Unsigned  n_bits=16  bin_pt=0  align_bp=on  dbl_ovrd=off  block_type=logical
      settings: xl_area=[1 1 0 1 0 0 0]  block_version=8.2-EVAL
  Logical1 : xbsIndex_r4/Logical  logical_function=AND  inputs=2  en=off  latency=1  precision=Full  arith_type=Unsigned  n_bits=16  bin_pt=0  align_bp=on  dbl_ovrd=off  block_type=logical
      settings: xl_area=[1 1 0 1 0 0 0]  block_version=8.2-EVAL
  Out1 : Outport
  wires:
  Logical1/1 -> Out1/1
  Logical/1 -> Logical1/2
  Inverter/1 -> Logical1/1
  Delay3/1 -> Logical/2
  In1/1 -> Delay3/1, Inverter/1, Logical/1

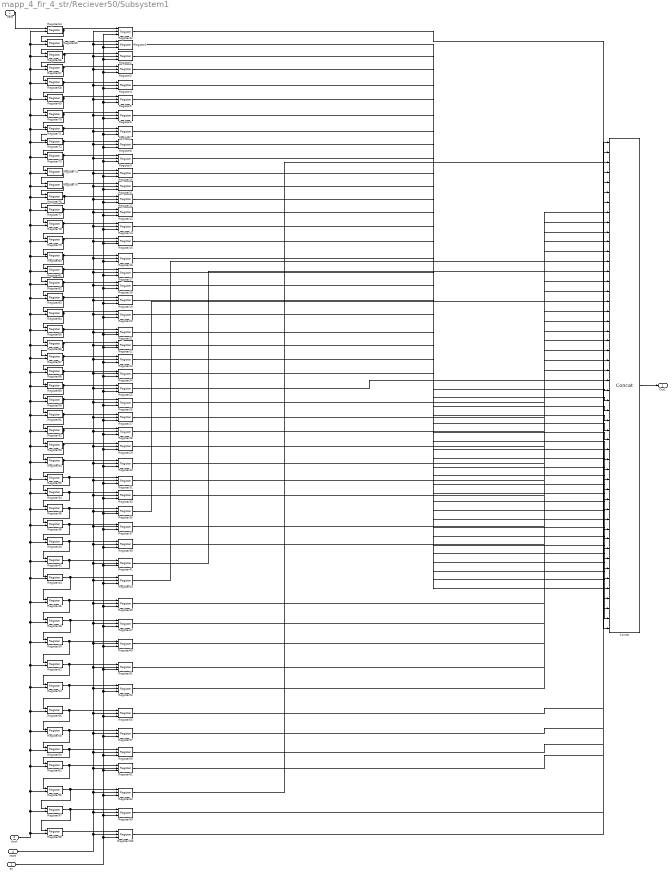
== system mapp_4_fir_4_str/Reciever50/Subsystem1 ==
  data : Inport
  en : Inport  Port=2
  clock : Inport  Port=3
  reset : Inport  Port=4
  Concat : xbsIndex_r4/Concat  num_inputs=50  dbl_ovrd=off  block_type=concat
      settings: block_version=8.2-EVAL
  Register{1..33,35,37,39,41,43,45,47,49,51,53,55,57,59,61,63,99..100} (50 alike) : xbsIndex_r4/Register  init=0  rst=on  en=on  dbl_ovrd=off  block_type=register
      settings: xl_area=[1 1 0 0 0 0 0]  block_version=8.2-EVAL
  Register{34,36,38,40,42,44,46,48,50,52,54,56,58,60,62,64..98} (50 alike) : xbsIndex_r4/Register  init=0  rst=off  en=on  dbl_ovrd=off  block_type=register
      settings: xl_area=[1 1 0 0 0 0 0]  block_version=8.2-EVAL
  Out1 : Outport
  wires:
  Concat/1 -> Out1/1
  Register100/1 -> Concat/1
  Register99/1 -> Concat/2
  Register98/1 -> Register100/1
  Register97/1 -> Register99/1, Register98/1
  clock/1 -> Register90/2, Register72/2, Register66/2, Register65/2, Register64/2, Register67/2, Register68/2, Register69/2, Register70/2, Register71/2, Register73/2, Register74/2, Register75/2, Register76/2, Register77/2, Register78/2, Register79/2, Register80/2, Register81/2, Register82/2, Register83/2, Register84/2, Register85/2, Register86/2, Register87/2, Register88/2, Register89/2, Register91/2, Register92/2, Register93/2, Register94/2, Register95/2, Register34/2, Register36/2, Register38/2, Register40/2, Register42/2, Register44/2, Register46/2, Register48/2, Register50/2, Register52/2, Register54/2, Register56/2, Register58/2, Register60/2, Register62/2, Register96/2, Register97/2, Register98/2
  Register94/1 -> Register30/1, Register95/1
  Register93/1 -> Register29/1, Register94/1
  Register92/1 -> Register28/1, Register93/1
  Register91/1 -> Register27/1, Register92/1
  Register90/1 -> Register26/1, Register91/1
  Register89/1 -> Register25/1, Register90/1
  Register88/1 -> Register24/1, Register89/1
  Register87/1 -> Register23/1, Register88/1
  Register86/1 -> Register22/1, Register87/1
  Register85/1 -> Register21/1, Register86/1
  Register84/1 -> Register20/1, Register85/1
  Register83/1 -> Register19/1, Register84/1
  Register82/1 -> Register18/1, Register83/1
  Register81/1 -> Register17/1, Register82/1
  Register80/1 -> Register16/1, Register81/1
  Register79/1 -> Register15/1, Register80/1
  Register78/1 -> Register14/1, Register79/1
  Register77/1 -> Register13/1, Register78/1
  Register76/1 -> Register12/1, Register77/1
  Register75/1 -> Register11/1, Register76/1
  Register74/1 -> Register10/1, Register75/1
  Register73/1 -> Register9/1, Register74/1
  Register72/1 -> Register8/1, Register73/1
  Register71/1 -> Register7/1, Register72/1
  Register70/1 -> Register6/1, Register71/1
  Register69/1 -> Register5/1, Register70/1
  Register68/1 -> Register4/1, Register69/1
  Register67/1 -> Register3/1, Register68/1
  Register66/1 -> Register2/1, Register67/1
  Register65/1 -> Register1/1, Register66/1
  data/1 -> Register64/1
  Register64/1 -> Register32/1, Register65/1
  Register95/1 -> Register31/1, Register34/1
  en/1 -> Register63/3, Register61/3, Register59/3, Register57/3, Register55/3, Register53/3, Register51/3, Register49/3, Register47/3, Register45/3, Register43/3, Register41/3, Register39/3, Register37/3, Register35/3, Register3/3, Register2/3, Register32/3, Register1/3, Register4/3, Register5/3, Register6/3, Register7/3, Register8/3, Register9/3, Register10/3, Register11/3, Register12/3, Register13/3, Register14/3, Register15/3, Register16/3, Register17/3, Register18/3, Register19/3, Register20/3, Register21/3, Register22/3, Register23/3, Register24/3, Register25/3, Register26/3, Register27/3, Register28/3, Register29/3, Register30/3, Register31/3, Register33/3, Register99/3, Register100/3
  reset/1 -> Register53/2, Register41/2, Register30/2, Register29/2, Register32/2, Register1/2, Register2/2, Register3/2, Register4/2, Register5/2, Register6/2, Register7/2, Register8/2, Register9/2, Register10/2, Register11/2, Register12/2, Register13/2, Register14/2, Register15/2, Register16/2, Register17/2, Register18/2, Register19/2, Register20/2, Register21/2, Register22/2, Register23/2, Register24/2, Register25/2, Register26/2, Register27/2, Register28/2, Register31/2, Register33/2, Register35/2, Register37/2, Register39/2, Register43/2, Register45/2, Register47/2, Register49/2, Register51/2, Register55/2, Register57/2, Register59/2, Register61/2, Register63/2, Register99/2, Register100/2
  Register34/1 -> Register33/1, Register36/1
  Register36/1 -> Register35/1, Register38/1
  Register38/1 -> Register37/1, Register40/1
  Register40/1 -> Register39/1, Register42/1
  Register42/1 -> Register41/1, Register44/1
  Register44/1 -> Register43/1, Register46/1
  Register46/1 -> Register45/1, Register48/1
  Register48/1 -> Register47/1, Register50/1
  Register50/1 -> Register49/1, Register52/1
  Register52/1 -> Register51/1, Register54/1
  Register54/1 -> Register53/1, Register56/1
  Register56/1 -> Register55/1, Register58/1
  Register58/1 -> Register57/1, Register60/1
  Register60/1 -> Register59/1, Register62/1
  Register62/1 -> Register61/1, Register96/1
  Register96/1 -> Register63/1, Register97/1
  Register63/1 -> Concat/3
  Register61/1 -> Concat/4
  Register59/1 -> Concat/5
  Register57/1 -> Concat/6
  Register55/1 -> Concat/7
  Register53/1 -> Concat/8
  Register51/1 -> Concat/9
  Register49/1 -> Concat/10
  Register47/1 -> Concat/11
  Register45/1 -> Concat/12
  Register43/1 -> Concat/13
  Register41/1 -> Concat/14
  Register39/1 -> Concat/15
  Register37/1 -> Concat/16
  Register35/1 -> Concat/17
  Register33/1 -> Concat/18
  Register31/1 -> Concat/19
  Register30/1 -> Concat/20
  Register29/1 -> Concat/21
  Register28/1 -> Concat/22
  Register27/1 -> Concat/23
  Register26/1 -> Concat/24
  Register25/1 -> Concat/25
  Register24/1 -> Concat/26
  Register23/1 -> Concat/27
  Register22/1 -> Concat/28
  Register21/1 -> Concat/29
  Register20/1 -> Concat/30
  Register19/1 -> Concat/31
  Register18/1 -> Concat/32
  Register17/1 -> Concat/33
  Register16/1 -> Concat/34
  Register15/1 -> Concat/35
  Register14/1 -> Concat/36
  Register13/1 -> Concat/37
  Register12/1 -> Concat/38
  Register11/1 -> Concat/39
  Register10/1 -> Concat/40
  Register9/1 -> Concat/41
  Register8/1 -> Concat/42
  Register7/1 -> Concat/43
  Register6/1 -> Concat/44
  Register5/1 -> Concat/45
  Register4/1 -> Concat/46
  Register3/1 -> Concat/47
  Register2/1 -> Concat/48
  Register1/1 -> Concat/49
  Register32/1 -> Concat/50

== system mapp_4_fir_4_str/Reciever50/Z1 ==
  In1 : Inport
  Delay3 : xbsIndex_r4/Delay  rst=off  infoeditControl=Selection of Reset will increase slice count due to use of real FFs and instead of SRLs  en=off  latency=1  reg_retiming=on  dbl_ovrd=off  block_type=delay
      settings: infoedit=Hardware notes: A delay line is a chain, each link of which is an SRL16 followed by a flip-flop. If register retiming is enabled, the delay line is a chain of flip-flops.  xl_area=[1 1 0 0 0 0 0]  block_version=8.2-EVAL
  Inverter : xbsIndex_r4/Inverter  en=off  latency=1  dbl_ovrd=off  block_type=inv
      settings: xl_area=[1 1 0 0 0 0 0]  block_version=8.2-EVAL
  Logical : xbsIndex_r4/Logical  logical_function=XOR  inputs=2  en=off  latency=1  precision=Full  arith_type=Unsigned  n_bits=16  bin_pt=0  align_bp=on  dbl_ovrd=off  block_type=logical
      settings: xl_area=[1 1 0 1 0 0 0]  block_version=8.2-EVAL
  Logical1 : xbsIndex_r4/Logical  logical_function=AND  inputs=2  en=off  latency=1  precision=Full  arith_type=Unsigned  n_bits=16  bin_pt=0  align_bp=on  dbl_ovrd=off  block_type=logical
      settings: xl_area=[1 1 0 1 0 0 0]  block_version=8.2-EVAL
  Out1 : Outport
  wires:
  In1/1 -> Logical/1, Inverter/1, Delay3/1
  Delay3/1 -> Logical/2
  Inverter/1 -> Logical1/1
  Logical/1 -> Logical1/2
  Logical1/1 -> Out1/1

== system mapp_4_fir_4_str/Svertka6/Count ==
  In1 : Inport
  start : Inport  Port=2
  Constant1 : xbsIndex_r4/Constant  const=1  gui_display_data_type=Fixed-point  arith_type=Boolean  n_bits=5  bin_pt=0  preci_type=Single  exp_width=8  frac_width=24  explicit_period=off  period=1  equ=P=C  opselect=C  inp2=PCIN>>17  opr=+  inp1=P  carry=CIN  dbl_ovrd=off  block_type=constant
      settings: block_version=VER_STRING_GOES_HERE
  Counter1 : xbsIndex_r4/Counter  cnt_type=Free Running  cnt_to=1  operation=Up  start_count=0  cnt_by_val=1  arith_type=Unsigned  n_bits=10  bin_pt=0  load_pin=off  rst=off  en=on  explicit_period=on  period=1  use_behavioral_HDL=off  implementation=Fabric  use_rpm=off  dbl_ovrd=off  block_type=counter
      settings: block_version=8.2.02
  Counter2 : xbsIndex_r4/Counter  cnt_type=Free Running  cnt_to=num_point_256*num_str_12*1 - 1  operation=Up  start_count=0  cnt_by_val=1  arith_type=Unsigned  n_bits=10  bin_pt=0  load_pin=off  rst=off  en=on  explicit_period=on  period=1  use_behavioral_HDL=off  implementation=Fabric  use_rpm=off  dbl_ovrd=off  block_type=counter
      settings: block_version=8.2.02
  Delay2 : xbsIndex_r4/Delay  rst=off  infoeditControl=Selection of Reset will increase slice count due to use of real FFs and instead of SRLs  en=off  latency=1  reg_retiming=on  dbl_ovrd=off  block_type=delay
      settings: xl_area=[2 4 0 4 0 0 0]  block_version=8.2-EVAL
  Register6 : xbsIndex_r4/Register  init=0  rst=off  en=on  dbl_ovrd=off  block_type=register
  Relational1 : xbsIndex_r4/Relational  mode=a=b  op_type=Bool  en=off  latency=1  dbl_ovrd=off  block_type=relational
      settings: xl_area=[4 1 0 7 0 0 0]  block_version=VER_STRING_GOES_HERE
  Out1 : Outport
  wires:
  start/1 -> Delay2/1
  Delay2/1 -> Counter1/1
  Counter2/1 -> Out1/1
  In1/1 -> Relational1/2
  Register6/1 -> Counter2/1
  Relational1/1 -> Register6/2
  Constant1/1 -> Register6/1
  Counter1/1 -> Relational1/1

== system mapp_4_fir_4_str/Svertka6/accum_0 ==
  In1 : Inport
  sig : Inport  Port=2
  coeff : Inport  Port=3
  reset : Inport  Port=4
  Accum_fl : Subsystem
  Constant47 : xbsIndex_r4/Constant  const=3  gui_display_data_type=Fixed-point  arith_type=Unsigned  n_bits=2  bin_pt=0  preci_type=Single  exp_width=8  frac_width=24  explicit_period=on  period=1  equ=P=C  opselect=C  inp2=PCIN>>17  opr=+  inp1=P  carry=CIN  dbl_ovrd=off  block_type=constant
      settings: block_version=VER_STRING_GOES_HERE
  Constant48 : xbsIndex_r4/Constant  const=0  gui_display_data_type=Fixed-point  arith_type=Unsigned  n_bits=2  bin_pt=0  preci_type=Single  exp_width=8  frac_width=24  explicit_period=on  period=1  equ=P=C  opselect=C  inp2=PCIN>>17  opr=+  inp1=P  carry=CIN  dbl_ovrd=off  block_type=constant
      settings: block_version=VER_STRING_GOES_HERE
  Constant49 : xbsIndex_r4/Constant  const=1  gui_display_data_type=Fixed-point  arith_type=Unsigned  n_bits=2  bin_pt=0  preci_type=Single  exp_width=8  frac_width=24  explicit_period=on  period=1  equ=P=C  opselect=C  inp2=PCIN>>17  opr=+  inp1=P  carry=CIN  dbl_ovrd=off  block_type=constant
      settings: block_version=VER_STRING_GOES_HERE
  Constant50 : xbsIndex_r4/Constant  const=2  gui_display_data_type=Fixed-point  arith_type=Unsigned  n_bits=2  bin_pt=0  preci_type=Single  exp_width=8  frac_width=24  explicit_period=on  period=1  equ=P=C  opselect=C  inp2=PCIN>>17  opr=+  inp1=P  carry=CIN  dbl_ovrd=off  block_type=constant
      settings: block_version=VER_STRING_GOES_HERE
  Convert : xbsIndex_r4/Convert  gui_display_data_type=Boolean  arith_type=Boolean  n_bits=16  bin_pt=14  float_type=Single  exp_bits=8  fraction_bits=24  quantization=Truncate  overflow=Wrap  en=off  latency=0  pipeline=off  dbl_ovrd=off  block_type=convert
  Delay{1,127,130,138,140,280} (6 alike) : xbsIndex_r4/Delay  rst=off  infoeditControl=Selection of Reset will increase slice count due to use of real FFs and instead of SRLs  en=off  latency=1  reg_retiming=off  dbl_ovrd=off  block_type=delay
  Delay129 : xbsIndex_r4/Delay  rst=off  infoeditControl=Selection of Reset will increase slice count due to use of real FFs and instead of SRLs  en=off  latency=24  reg_retiming=off  dbl_ovrd=off  block_type=delay
  Delay131 : xbsIndex_r4/Delay  rst=off  infoeditControl=Selection of Reset will increase slice count due to use of real FFs and instead of SRLs  en=off  latency=2  reg_retiming=off  dbl_ovrd=off  block_type=delay
  Delay135 : xbsIndex_r4/Delay  rst=off  infoeditControl=Selection of Reset will increase slice count due to use of real FFs and instead of SRLs  en=off  latency=6  reg_retiming=off  dbl_ovrd=off  block_type=delay
  Delay136 : xbsIndex_r4/Delay  rst=off  infoeditControl=Selection of Reset will increase slice count due to use of real FFs and instead of SRLs  en=off  latency=42  reg_retiming=off  dbl_ovrd=off  block_type=delay
  Logical{34..37} (4 alike) : xbsIndex_r4/Logical  logical_function=AND  inputs=2  en=off  latency=0  precision=Full  arith_type=Unsigned  n_bits=16  bin_pt=0  align_bp=on  dbl_ovrd=off  block_type=logical
  Mult9 : xbsIndex_r4/Mult  precision=Full  arith_type="Signed  (2's comp)"  n_bits=16  bin_pt=14  quantization=Truncate  overflow=Wrap  en=off  latency=6  use_behavioral_HDL=off  opt=Speed  use_embedded=on  optimum_pipeline=off  pipeline=on  dbl_ovrd=off  use_rpm=on  placement_style=Triangular  block_type=mult
  Register{82..85} (4 alike) : xbsIndex_r4/Register  init=0  rst=off  en=on  dbl_ovrd=off  block_type=register
  Register87 : xbsIndex_r4/Register  init=0  rst=off  en=off  dbl_ovrd=off  block_type=register
  Relational{45,47..49} (4 alike) : xbsIndex_r4/Relational  mode=a=b  op_type=Bool  en=off  latency=1  dbl_ovrd=off  block_type=relational
  Slice1 : xbsIndex_r4/Slice  nbits=8  boolean_output=off  mode=Lower Bit Location + Width  bit1=0  base1=MSB of Input  bit0=0  base0=LSB of Input  dbl_ovrd=off  block_type=slice
  Slice12 : xbsIndex_r4/Slice  nbits=2  boolean_output=off  mode=Upper Bit Location + Width  bit1=0  base1=MSB of Input  bit0=0  base0=LSB of Input  dbl_ovrd=off  block_type=slice
  Slice38 : xbsIndex_r4/Slice  nbits=1  boolean_output=off  mode=Lower Bit Location + Width  bit1=0  base1=MSB of Input  bit0=7  base0=LSB of Input  dbl_ovrd=off  block_type=slice
  en14 : Subsystem
  Out1 : Outport
  Out2 : Outport  Port=2
  Out3 : Outport  Port=3
  Out4 : Outport  Port=4
  wires:
  Delay1/1 -> Convert/1
  Convert/1 -> Logical34/2, Logical35/2, Logical36/2, Logical37/2
  Slice1/1 -> Accum_fl/1(addr_256)
  en14/1(Out1) -> Delay129/1
  Accum_fl/1(sig_out) -> Register82/1, Register83/1, Register84/1, Register85/1
  Delay129/1 -> Delay1/1
  Register84/1 -> Out3/1
  sig/1 -> Delay130/1
  Logical34/1 -> Register82/2
  Slice12/1 -> Delay136/1
  Delay140/1 -> Mult9/2
  Slice38/1 -> en14/1(In1)
  Logical36/1 -> Register84/2
  Delay138/1 -> Mult9/1
  Logical37/1 -> Register85/2
  Relational47/1 -> Logical35/1
  Constant50/1 -> Relational47/2
  Delay135/1 -> Register87/1
  Relational45/1 -> Logical34/1
  coeff/1 -> Delay140/1
  Relational48/1 -> Logical36/1
  Relational49/1 -> Logical37/1
  Register83/1 -> Out2/1
  Constant49/1 -> Relational45/2
  In1/1 -> Delay280/1
  Constant48/1 -> Relational49/2
  Register85/1 -> Out4/1
  Logical35/1 -> Register83/2
  Delay280/1 -> Slice38/1, Slice12/1, Slice1/1
  Delay130/1 -> Delay131/1
  Delay131/1 -> Delay138/1
  Register82/1 -> Out1/1
  Constant47/1 -> Relational48/2
  Register87/1 -> Accum_fl/2(sig)
  Delay127/1 -> Delay135/1
  Mult9/1 -> Delay127/1
  Delay136/1 -> Relational49/1, Relational48/1, Relational47/1, Relational45/1
  reset/1 -> Accum_fl/3(reset)
